simulink model "L0606"  (Simulink 9.1)
settings: Solver=VariableStepAuto  StartTime=0.0  StopTime=10.0  RelTol=1e-3
settings Model: Creator=Asus  LastModifiedBy=Asus
settings DataIOCC: SaveFormat=Dataset
settings OptimizationCC: LifeSpan=auto
settings DebuggingCC: UnderspecifiedInitializationDetection=Simplified  MergeDetectMultiDrivingBlocksExec=error  SFUnexpectedBacktrackingDiag=error  SFNoUnconditionalDefaultTransitionDiag=error  SFExecutionAtInitializationDiag=warning
settings HardwareCC: ProdBitPerPointer=64  ProdBitPerSizeT=64  ProdBitPerPtrDiffT=64  ProdLargestAtomicFloat=Float  ProdIntDivRoundTo=Zero  ProdEndianess=LittleEndian  ProdWordSize=64  ProdHWDeviceType=Intel->x86-64 (Windows64)
settings ModelReferenceCC: PropagateSignalLabelsOutOfModel=on
settings CodeAppCC: StateflowObjectComments=off
settings GRTTargetCC: TargetLangStandard=C99 (ISO)  CombineOutputUpdateFcns=on  GRTInterface=off
settings ConfigComp: CovMetricSettings=dwe  CovHtmlReporting=off  CovSaveCumulativeToWorkspaceVar=off  CovSaveSingleToWorkspaceVar=off  CovExternalEMLEnable=on

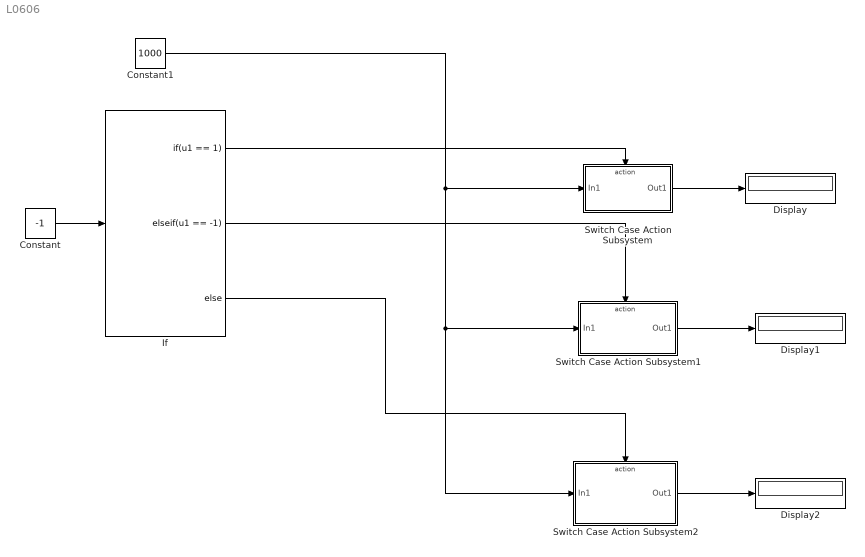
== system L0606 ==
  Constant : Constant  Value=-1
  Constant1 : Constant  Value=1000
  Display : Display
  Display1 : Display
  Display2 : Display
  If : If  IfExpression=u1 == 1  ElseIfExpressions=u1 == -1
  Switch Case Action Subsystem : Subsystem  TreatAsAtomicUnit=on
  Switch Case Action Subsystem1 : Subsystem  TreatAsAtomicUnit=on
  Switch Case Action Subsystem2 : Subsystem  TreatAsAtomicUnit=on
  wires:
  Constant/1 -> If/1
  If/2 -> Switch Case Action Subsystem1/Action
  If/3 -> Switch Case Action Subsystem2/Action
  Switch Case Action Subsystem2/1(Out1) -> Display2/1
  If/1 -> Switch Case Action Subsystem/Action
  Switch Case Action Subsystem1/1(Out1) -> Display1/1
  Constant1/1 -> Switch Case Action Subsystem2/1(In1), Switch Case Action Subsystem1/1(In1), Switch Case Action Subsystem/1(In1)
  Switch Case Action Subsystem/1(Out1) -> Display/1

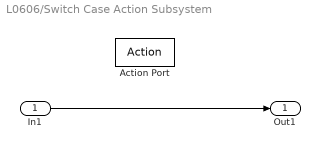
== system L0606/Switch Case Action Subsystem ==
  In1 : Inport
  Action Port : ActionPort  ActionType=then
  Out1 : Outport
  wires:
  In1/1 -> Out1/1

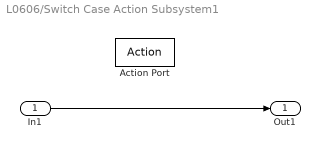
== system L0606/Switch Case Action Subsystem1 ==
  In1 : Inport
  Action Port : ActionPort  ActionType=elseif
  Out1 : Outport
  wires:
  In1/1 -> Out1/1

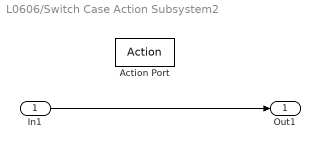
== system L0606/Switch Case Action Subsystem2 ==
  In1 : Inport
  Action Port : ActionPort  ActionType=else
  Out1 : Outport
  wires:
  In1/1 -> Out1/1
